simulink model "Frequency_Domain_Corrected_PN_Guidance"  (R2025b)
settings: Solver=VariableStepAuto  StartTime=0.0  StopTime=Inf  RelTol=1e-3  EnableMultiTasking=on
values from neighbouring files (symbols this model uses):
  a_cmax = 600    [APN.m]    (also in PN.m; ZMD_PN.m)
  a_Tmax = 200    [APN.m]    (also in PN.m; ZMD_PN.m)
  h = conv(conv([0.1 1],[0.1 1]),[0.1 1])    [APN.m]    (also in PN.m; ZMD_PN.m; thesis_guidance_sim.m = [1, 0.15, 0.0225])
  intercept_time = 10    [APN.m]    (also in PN.m; ZMD_PN.m)
  Mode = 2    [APN.m]    (also in PN.m = 1; ZMD_PN.m = 3)
  N = 5    [APN.m]    (also in PN.m; ZMD_PN.m; thesis_guidance_sim.m = N_or_table(iz,it))
  tau = 0.3    [APN.m]    (also in PN.m; ZMD_PN.m; thesis_guidance_sim.m = 0.1)
  Ts_guidance = 0.001    [APN.m]    (also in PN.m; ZMD_PN.m; thesis_guidance_sim.m = 0.05)
  v_cl = 1000    [APN.m]    (also in PN.m; ZMD_PN.m)
  w_n = 10    [APN.m]    (also in PN.m; ZMD_PN.m)
  zeta = 0.5    [APN.m]    (also in PN.m; ZMD_PN.m; thesis_guidance_sim.m = 0.7)
undefined symbols (not defined in the file or in its folder): w_T, w_z
libraries: simulink x4
Description:
  | PN、APN、ZMD-PN、Scheduled-Gain控制，二维导弹拦截迂回机动目标仿真
settings Model: Creator=杨智豪  LastModifiedBy=杨智豪
settings DataIOCC: SaveOutput=off  SignalLogging=off  DSMLogging=off  SaveTime=off  ReturnWorkspaceOutputs=off

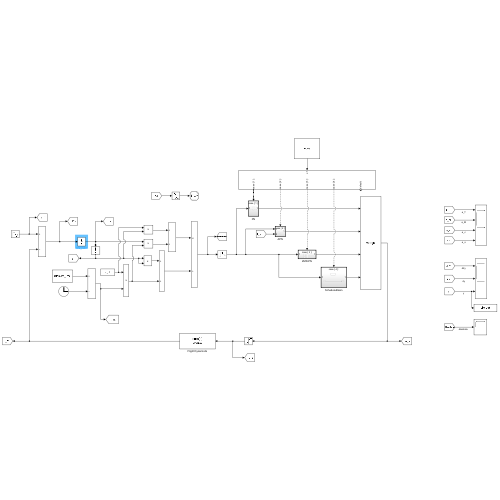
[thumbnail: Simulink's stored preview of the top-level diagram]
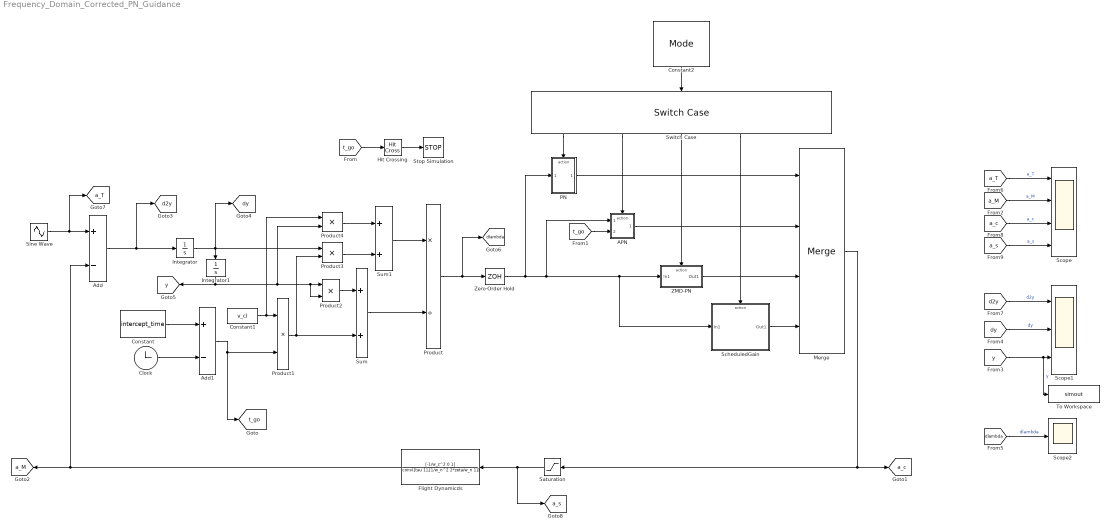
== system Frequency_Domain_Corrected_PN_Guidance ==
  APN : Subsystem
  Add : Sum  Inputs=+-
  Add1 : Sum  Inputs=+-
  Clock : Clock
  Constant : Constant  Value=intercept_time
  Constant1 : Constant  Value=v_cl
  Constant2 : Constant  Value=Mode
  Flight Dynamicds : TransferFcn  Numerator=[-1/w_z^2 0 1]  Denominator=conv([tau 1],[1/w_n^2 2*zeta/w_n 1])
  Hit Crossing : HitCross  HitCrossingDirection=falling
  Integrator : Integrator  InitialCondition=-1000
  Integrator1 : Integrator
  Merge : Merge  Inputs=4
  PN : Subsystem
  Product : Product  Inputs=*/
  Product{1..4} (4 alike) : Product
  Saturation : Saturate  UpperLimit=a_cmax  LowerLimit=-a_cmax
  ScheduledGain : Subsystem
  Scope : Scope  NumInputPorts=4
      settings: ActiveDisplayYMinimum=-846.61582392011235  ActiveDisplayYMaximum=816.29400987499253
  Scope1 : Scope  NumInputPorts=3
      settings: ActiveDisplayYMinimum=-12.158424024464928  ActiveDisplayYMaximum=-3.8394674734413305  DataLoggingVariableName=y
  Scope2 : Scope
      settings: ActiveDisplayYMinimum=-310.05048506745004  ActiveDisplayYMaximum=2516.5257182111445  DataLoggingVariableName=ScopeData2
  Sine Wave : Sin  Amplitude=a_Tmax  Frequency=w_T  Phase=pi/2  SampleTime=0
  Stop Simulation : Stop
  Sum : Sum
  Sum1 : Sum
  Switch Case : SwitchCase  CaseConditions={1, 2, 3, 4}
  To Workspace : ToWorkspace  VariableName=simout  SampleTime=-1
  ZMD-PN : Subsystem  TreatAsAtomicUnit=on
  Zero-Order Hold : ZeroOrderHold  SampleTime=Ts_guidance
  tag scope: a_M=global, a_T=global, a_c=global, a_s=global, d2y=global, dlambda=global, dy=global, t_go=global, y=global
  wires:
  Sine Wave/1 -> [a_T], Add/1
  Add/1 -> [d2y], Integrator/1
  Integrator/1 -> Product3/1, Integrator1/1, [dy]
  Clock/1 -> Add1/2
  Constant/1 -> Add1/1
  Flight Dynamicds/1 -> Add/2, [a_M]
  Saturation/1 -> [a_s], Flight Dynamicds/1
  Product/1 -> [dlambda], Zero-Order Hold/1
  Integrator1/1 -> Product4/2, Product2/2, Product2/1, [y]
  Constant1/1 -> Product4/1, Product1/1
  Sum/1 -> Product/2
  Product1/1 -> Product3/2, Sum/2
  Product2/1 -> Sum/1
  Product4/1 -> Sum1/1
  Product3/1 -> Sum1/2
  Sum1/1 -> Product/1
  Zero-Order Hold/1 -> PN/1(In1), ScheduledGain/1(In1), ZMD-PN/1(In1), APN/1(In1)
  Switch Case/3 -> ZMD-PN/Action
  Constant2/1 -> Switch Case/1
  Switch Case/1 -> PN/Action
  [t_go] -> Hit Crossing/1
  Hit Crossing/1 -> Stop Simulation/1
  Switch Case/2 -> APN/Action
  Switch Case/4 -> ScheduledGain/Action
  APN/1(Out1) -> Merge/2
  ScheduledGain/1(Out1) -> Merge/4
  ZMD-PN/1(Out1) -> Merge/3
  PN/1(Out1) -> Merge/1
  Merge/1 -> Saturation/1, [a_c]
  [t_go] -> APN/2(In2)
  [a_c] -> Scope/3  "a_c"
  [a_M] -> Scope/2  "a_M"
  [y] -> To Workspace/1, Scope1/3  "y"
  [dy] -> Scope1/2  "dy"
  [d2y] -> Scope1/1  "d2y"
  [dlambda] -> Scope2/1  "dlambda"
  [a_T] -> Scope/1  "a_T"
  [a_s] -> Scope/4  "a_s"
  Add1/1 -> [t_go], Product1/2

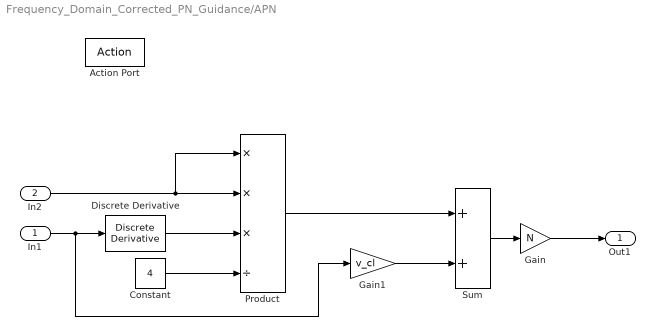
== system Frequency_Domain_Corrected_PN_Guidance/APN ==
  In1 : Inport
  In2 : Inport  Port=2
  Action Port : ActionPort  InitializeStates=reset  ActionPortLabel=case [ 2 ]:
  Constant : Constant  Value=4
  Discrete Derivative : simulink/Discrete/Discrete Derivative  gainval=1.0  ICPrevScaledInput=0.0  OutMin=[]  OutMax=[]  OutDataType=fixdt(1, 16)  OutScaling=2^-10  DoSatur=off
  Gain : Gain  Gain=N
  Gain1 : Gain  Gain=v_cl
  Product : Product  Inputs=***/
  Sum : Sum
  Out1 : Outport
  wires:
  In2/1 -> Product/1, Product/2
  In1/1 -> Gain1/1, Discrete Derivative/1
  Discrete Derivative/1 -> Product/3
  Constant/1 -> Product/4
  Gain/1 -> Out1/1
  Sum/1 -> Gain/1
  Product/1 -> Sum/1
  Gain1/1 -> Sum/2

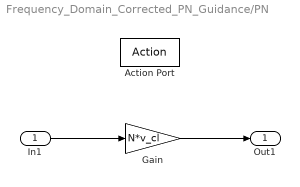
== system Frequency_Domain_Corrected_PN_Guidance/PN ==
  In1 : Inport
  Action Port : ActionPort  InitializeStates=reset  ActionPortLabel=case [ 1 ]:
  Gain : Gain  Gain=N*v_cl
  Out1 : Outport
  wires:
  In1/1 -> Gain/1
  Gain/1 -> Out1/1

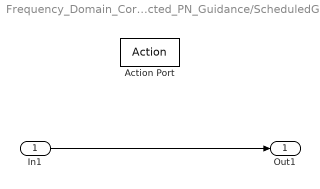
== system Frequency_Domain_Corrected_PN_Guidance/ScheduledGain ==
  In1 : Inport
  Action Port : ActionPort  InitializeStates=reset  ActionPortLabel=case [ 4 ]:
  Out1 : Outport
  wires:
  In1/1 -> Out1/1

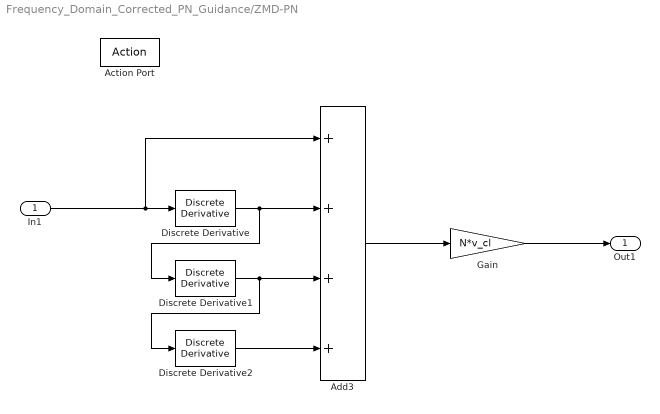
== system Frequency_Domain_Corrected_PN_Guidance/ZMD-PN ==
  In1 : Inport
  Action Port : ActionPort  InitializeStates=reset  ActionPortLabel=case [ 3 ]:
  Add3 : Sum  Inputs=++++
  Discrete Derivative : simulink/Discrete/Discrete Derivative  gainval=h(3)  ICPrevScaledInput=0.0  OutMin=[]  OutMax=[]  OutDataType=fixdt(1, 16)  OutScaling=2^-10  DoSatur=off
  Discrete Derivative1 : simulink/Discrete/Discrete Derivative  gainval=h(2)  ICPrevScaledInput=0.0  OutMin=[]  OutMax=[]  OutDataType=fixdt(1, 16)  OutScaling=2^-10  DoSatur=off
  Discrete Derivative2 : simulink/Discrete/Discrete Derivative  gainval=h(1)  ICPrevScaledInput=0.0  OutMin=[]  OutMax=[]  OutDataType=fixdt(1, 16)  OutScaling=2^-10  DoSatur=off
  Gain : Gain  Gain=N*v_cl
  Out1 : Outport
  wires:
  In1/1 -> Add3/1, Discrete Derivative/1
  Discrete Derivative/1 -> Add3/2, Discrete Derivative1/1
  Add3/1 -> Gain/1
  Gain/1 -> Out1/1
  Discrete Derivative2/1 -> Add3/4
  Discrete Derivative1/1 -> Discrete Derivative2/1, Add3/3
